simulink model "MATE_9LevelDrive_LowHarmonicRectifier"  (R2024b)
settings: Solver=FixedStepDiscrete  StartTime=0.0  StopTime=1  FixedStep=Ts  RelTol=1e-3
PostLoadFcn:
  | Ts=25e-6; initDrive9Level;Rsnu=30; Csnu=3e-6;Ron=0.01;Roff=1e6; Vf=2;
InitFcn:
  | Ts=25e-6; initDrive9Level;Rsnu=30; Csnu=3e-6;Ron=0.01;Roff=1e6; Vf=2;
values from neighbouring files (symbols this model uses):
  Lbase = Zbase/wbase    (= 0.0044902914611)    [initDrive9Level.m]
  Rgnd_rectifier = 1e4    (= 10000)    [initDrive9Level.m]
  T_2wind_ratio = 0.2677    [initDrive9Level.m]
  T_Lpu = Ltot_pu*9/10    (= 0.036)    [initDrive9Level.m]
  T_Lpu_pri = Ltot_pu/10    (= 0.004)    [initDrive9Level.m]
  T_Rpu = Rtot_pu*9/10    (= 0.009)    [initDrive9Level.m]
  T_Rpu_pri = Rtot_pu/10    (= 0.001)    [initDrive9Level.m]
  T_Vpri = 3000    [initDrive9Level.m]
  T_Vpri_15comp = 1.1168    [initDrive9Level.m]
  T_Vsec = 920    [initDrive9Level.m]
  Zbase = T_Vsec*T_Vsec/T_Pbase    (= 1.6928)    [initDrive9Level.m]
undefined symbols (not defined in the file or in its folder): DiscIntNeverNeededParam, gcbh, sps_rtmsupport
libraries: fl_lib x192, ee_lib x105, simetranss x26, nesl_utility x21
(part 4 of 5)

== system MATE_9LevelDrive_LowHarmonicRectifier/Diode Bridge with snubber2/RCsnuber2 ==
  Capacitor : fl_lib/Electrical/Electrical Elements/Capacitor  c=Csnu F  r=0 Ohm  g=0 1/Ohm  i_specify=off  i_priority=None  i=0 A  i_nominal_specify=off  i_nominal_value=1  i_nominal_unit=A  v_specify=off  v_priority=None  v=0 V  v_nominal_specify=off  v_nominal_value=1  v_nominal_unit=V  vc_specify=off  vc_priority=High  vc=0 V  vc_nominal_specify=off  vc_nominal_value=1  vc_nominal_unit=V
  Resistor : fl_lib/Electrical/Electrical Elements/Resistor  R=Rsnu Ohm  i_specify=off  i_priority=None  i=0 A  i_nominal_specify=off  i_nominal_value=1  i_nominal_unit=A  v_specify=off  v_priority=None  v=0 V  v_nominal_specify=off  v_nominal_value=1  v_nominal_unit=V
  + : PMIOPort  Side=Left
  - : PMIOPort  Port=2  Side=Right
  connections:
  Resistor/RConn1 -- -/RConn1
  Capacitor/LConn1 -- +/RConn1
  Resistor/LConn1 -- Capacitor/RConn1

== system MATE_9LevelDrive_LowHarmonicRectifier/Diode Bridge with snubber2/RCsnuber3 ==
  Capacitor : fl_lib/Electrical/Electrical Elements/Capacitor  c=Csnu F  r=0 Ohm  g=0 1/Ohm  i_specify=off  i_priority=None  i=0 A  i_nominal_specify=off  i_nominal_value=1  i_nominal_unit=A  v_specify=off  v_priority=None  v=0 V  v_nominal_specify=off  v_nominal_value=1  v_nominal_unit=V  vc_specify=off  vc_priority=High  vc=0 V  vc_nominal_specify=off  vc_nominal_value=1  vc_nominal_unit=V
  Resistor : fl_lib/Electrical/Electrical Elements/Resistor  R=Rsnu Ohm  i_specify=off  i_priority=None  i=0 A  i_nominal_specify=off  i_nominal_value=1  i_nominal_unit=A  v_specify=off  v_priority=None  v=0 V  v_nominal_specify=off  v_nominal_value=1  v_nominal_unit=V
  + : PMIOPort  Side=Left
  - : PMIOPort  Port=2  Side=Right
  connections:
  Resistor/LConn1 -- Capacitor/RConn1
  Capacitor/LConn1 -- +/RConn1
  Resistor/RConn1 -- -/RConn1

== system MATE_9LevelDrive_LowHarmonicRectifier/Diode Bridge with snubber2/RCsnuber4 ==
  Capacitor : fl_lib/Electrical/Electrical Elements/Capacitor  c=Csnu F  r=0 Ohm  g=0 1/Ohm  i_specify=off  i_priority=None  i=0 A  i_nominal_specify=off  i_nominal_value=1  i_nominal_unit=A  v_specify=off  v_priority=None  v=0 V  v_nominal_specify=off  v_nominal_value=1  v_nominal_unit=V  vc_specify=off  vc_priority=High  vc=0 V  vc_nominal_specify=off  vc_nominal_value=1  vc_nominal_unit=V
  Resistor : fl_lib/Electrical/Electrical Elements/Resistor  R=Rsnu Ohm  i_specify=off  i_priority=None  i=0 A  i_nominal_specify=off  i_nominal_value=1  i_nominal_unit=A  v_specify=off  v_priority=None  v=0 V  v_nominal_specify=off  v_nominal_value=1  v_nominal_unit=V
  + : PMIOPort  Side=Left
  - : PMIOPort  Port=2  Side=Right
  connections:
  Resistor/LConn1 -- Capacitor/RConn1
  Capacitor/LConn1 -- +/RConn1
  Resistor/RConn1 -- -/RConn1

== system MATE_9LevelDrive_LowHarmonicRectifier/Diode Bridge with snubber2/RCsnuber5 ==
  Capacitor : fl_lib/Electrical/Electrical Elements/Capacitor  c=Csnu F  r=0 Ohm  g=0 1/Ohm  i_specify=off  i_priority=None  i=0 A  i_nominal_specify=off  i_nominal_value=1  i_nominal_unit=A  v_specify=off  v_priority=None  v=0 V  v_nominal_specify=off  v_nominal_value=1  v_nominal_unit=V  vc_specify=off  vc_priority=High  vc=0 V  vc_nominal_specify=off  vc_nominal_value=1  vc_nominal_unit=V
  Resistor : fl_lib/Electrical/Electrical Elements/Resistor  R=Rsnu Ohm  i_specify=off  i_priority=None  i=0 A  i_nominal_specify=off  i_nominal_value=1  i_nominal_unit=A  v_specify=off  v_priority=None  v=0 V  v_nominal_specify=off  v_nominal_value=1  v_nominal_unit=V
  + : PMIOPort  Side=Left
  - : PMIOPort  Port=2  Side=Right
  connections:
  Resistor/RConn1 -- -/RConn1
  Capacitor/LConn1 -- +/RConn1
  Resistor/LConn1 -- Capacitor/RConn1

== system MATE_9LevelDrive_LowHarmonicRectifier/Diode Bridge with snubber3/RCsnuber ==
  Capacitor : fl_lib/Electrical/Electrical Elements/Capacitor  c=Csnu F  r=0 Ohm  g=0 1/Ohm  i_specify=off  i_priority=None  i=0 A  i_nominal_specify=off  i_nominal_value=1  i_nominal_unit=A  v_specify=off  v_priority=None  v=0 V  v_nominal_specify=off  v_nominal_value=1  v_nominal_unit=V  vc_specify=off  vc_priority=High  vc=0 V  vc_nominal_specify=off  vc_nominal_value=1  vc_nominal_unit=V
  Resistor : fl_lib/Electrical/Electrical Elements/Resistor  R=Rsnu Ohm  i_specify=off  i_priority=None  i=0 A  i_nominal_specify=off  i_nominal_value=1  i_nominal_unit=A  v_specify=off  v_priority=None  v=0 V  v_nominal_specify=off  v_nominal_value=1  v_nominal_unit=V
  + : PMIOPort  Side=Left
  - : PMIOPort  Port=2  Side=Right
  connections:
  Resistor/LConn1 -- Capacitor/RConn1
  Capacitor/LConn1 -- +/RConn1
  Resistor/RConn1 -- -/RConn1

== system MATE_9LevelDrive_LowHarmonicRectifier/Diode Bridge with snubber3/RCsnuber1 ==
  Capacitor : fl_lib/Electrical/Electrical Elements/Capacitor  c=Csnu F  r=0 Ohm  g=0 1/Ohm  i_specify=off  i_priority=None  i=0 A  i_nominal_specify=off  i_nominal_value=1  i_nominal_unit=A  v_specify=off  v_priority=None  v=0 V  v_nominal_specify=off  v_nominal_value=1  v_nominal_unit=V  vc_specify=off  vc_priority=High  vc=0 V  vc_nominal_specify=off  vc_nominal_value=1  vc_nominal_unit=V
  Resistor : fl_lib/Electrical/Electrical Elements/Resistor  R=Rsnu Ohm  i_specify=off  i_priority=None  i=0 A  i_nominal_specify=off  i_nominal_value=1  i_nominal_unit=A  v_specify=off  v_priority=None  v=0 V  v_nominal_specify=off  v_nominal_value=1  v_nominal_unit=V
  + : PMIOPort  Side=Left
  - : PMIOPort  Port=2  Side=Right
  connections:
  Resistor/RConn1 -- -/RConn1
  Capacitor/LConn1 -- +/RConn1
  Resistor/LConn1 -- Capacitor/RConn1

== system MATE_9LevelDrive_LowHarmonicRectifier/Diode Bridge with snubber3/RCsnuber2 ==
  Capacitor : fl_lib/Electrical/Electrical Elements/Capacitor  c=Csnu F  r=0 Ohm  g=0 1/Ohm  i_specify=off  i_priority=None  i=0 A  i_nominal_specify=off  i_nominal_value=1  i_nominal_unit=A  v_specify=off  v_priority=None  v=0 V  v_nominal_specify=off  v_nominal_value=1  v_nominal_unit=V  vc_specify=off  vc_priority=High  vc=0 V  vc_nominal_specify=off  vc_nominal_value=1  vc_nominal_unit=V
  Resistor : fl_lib/Electrical/Electrical Elements/Resistor  R=Rsnu Ohm  i_specify=off  i_priority=None  i=0 A  i_nominal_specify=off  i_nominal_value=1  i_nominal_unit=A  v_specify=off  v_priority=None  v=0 V  v_nominal_specify=off  v_nominal_value=1  v_nominal_unit=V
  + : PMIOPort  Side=Left
  - : PMIOPort  Port=2  Side=Right
  connections:
  Resistor/LConn1 -- Capacitor/RConn1
  Capacitor/LConn1 -- +/RConn1
  Resistor/RConn1 -- -/RConn1

== system MATE_9LevelDrive_LowHarmonicRectifier/Diode Bridge with snubber3/RCsnuber3 ==
  Capacitor : fl_lib/Electrical/Electrical Elements/Capacitor  c=Csnu F  r=0 Ohm  g=0 1/Ohm  i_specify=off  i_priority=None  i=0 A  i_nominal_specify=off  i_nominal_value=1  i_nominal_unit=A  v_specify=off  v_priority=None  v=0 V  v_nominal_specify=off  v_nominal_value=1  v_nominal_unit=V  vc_specify=off  vc_priority=High  vc=0 V  vc_nominal_specify=off  vc_nominal_value=1  vc_nominal_unit=V
  Resistor : fl_lib/Electrical/Electrical Elements/Resistor  R=Rsnu Ohm  i_specify=off  i_priority=None  i=0 A  i_nominal_specify=off  i_nominal_value=1  i_nominal_unit=A  v_specify=off  v_priority=None  v=0 V  v_nominal_specify=off  v_nominal_value=1  v_nominal_unit=V
  + : PMIOPort  Side=Left
  - : PMIOPort  Port=2  Side=Right
  connections:
  Resistor/RConn1 -- -/RConn1
  Capacitor/LConn1 -- +/RConn1
  Resistor/LConn1 -- Capacitor/RConn1

== system MATE_9LevelDrive_LowHarmonicRectifier/Diode Bridge with snubber3/RCsnuber4 ==
  Capacitor : fl_lib/Electrical/Electrical Elements/Capacitor  c=Csnu F  r=0 Ohm  g=0 1/Ohm  i_specify=off  i_priority=None  i=0 A  i_nominal_specify=off  i_nominal_value=1  i_nominal_unit=A  v_specify=off  v_priority=None  v=0 V  v_nominal_specify=off  v_nominal_value=1  v_nominal_unit=V  vc_specify=off  vc_priority=High  vc=0 V  vc_nominal_specify=off  vc_nominal_value=1  vc_nominal_unit=V
  Resistor : fl_lib/Electrical/Electrical Elements/Resistor  R=Rsnu Ohm  i_specify=off  i_priority=None  i=0 A  i_nominal_specify=off  i_nominal_value=1  i_nominal_unit=A  v_specify=off  v_priority=None  v=0 V  v_nominal_specify=off  v_nominal_value=1  v_nominal_unit=V
  + : PMIOPort  Side=Left
  - : PMIOPort  Port=2  Side=Right
  connections:
  Resistor/RConn1 -- -/RConn1
  Capacitor/LConn1 -- +/RConn1
  Resistor/LConn1 -- Capacitor/RConn1

== system MATE_9LevelDrive_LowHarmonicRectifier/Diode Bridge with snubber3/RCsnuber5 ==
  Capacitor : fl_lib/Electrical/Electrical Elements/Capacitor  c=Csnu F  r=0 Ohm  g=0 1/Ohm  i_specify=off  i_priority=None  i=0 A  i_nominal_specify=off  i_nominal_value=1  i_nominal_unit=A  v_specify=off  v_priority=None  v=0 V  v_nominal_specify=off  v_nominal_value=1  v_nominal_unit=V  vc_specify=off  vc_priority=High  vc=0 V  vc_nominal_specify=off  vc_nominal_value=1  vc_nominal_unit=V
  Resistor : fl_lib/Electrical/Electrical Elements/Resistor  R=Rsnu Ohm  i_specify=off  i_priority=None  i=0 A  i_nominal_specify=off  i_nominal_value=1  i_nominal_unit=A  v_specify=off  v_priority=None  v=0 V  v_nominal_specify=off  v_nominal_value=1  v_nominal_unit=V
  + : PMIOPort  Side=Left
  - : PMIOPort  Port=2  Side=Right
  connections:
  Resistor/LConn1 -- Capacitor/RConn1
  Capacitor/LConn1 -- +/RConn1
  Resistor/RConn1 -- -/RConn1

== system MATE_9LevelDrive_LowHarmonicRectifier/Diode Bridge with snubber4/RCsnuber ==
  Capacitor : fl_lib/Electrical/Electrical Elements/Capacitor  c=Csnu F  r=0 Ohm  g=0 1/Ohm  i_specify=off  i_priority=None  i=0 A  i_nominal_specify=off  i_nominal_value=1  i_nominal_unit=A  v_specify=off  v_priority=None  v=0 V  v_nominal_specify=off  v_nominal_value=1  v_nominal_unit=V  vc_specify=off  vc_priority=High  vc=0 V  vc_nominal_specify=off  vc_nominal_value=1  vc_nominal_unit=V
  Resistor : fl_lib/Electrical/Electrical Elements/Resistor  R=Rsnu Ohm  i_specify=off  i_priority=None  i=0 A  i_nominal_specify=off  i_nominal_value=1  i_nominal_unit=A  v_specify=off  v_priority=None  v=0 V  v_nominal_specify=off  v_nominal_value=1  v_nominal_unit=V
  + : PMIOPort  Side=Left
  - : PMIOPort  Port=2  Side=Right
  connections:
  Resistor/RConn1 -- -/RConn1
  Capacitor/LConn1 -- +/RConn1
  Resistor/LConn1 -- Capacitor/RConn1

== system MATE_9LevelDrive_LowHarmonicRectifier/Diode Bridge with snubber4/RCsnuber1 ==
  Capacitor : fl_lib/Electrical/Electrical Elements/Capacitor  c=Csnu F  r=0 Ohm  g=0 1/Ohm  i_specify=off  i_priority=None  i=0 A  i_nominal_specify=off  i_nominal_value=1  i_nominal_unit=A  v_specify=off  v_priority=None  v=0 V  v_nominal_specify=off  v_nominal_value=1  v_nominal_unit=V  vc_specify=off  vc_priority=High  vc=0 V  vc_nominal_specify=off  vc_nominal_value=1  vc_nominal_unit=V
  Resistor : fl_lib/Electrical/Electrical Elements/Resistor  R=Rsnu Ohm  i_specify=off  i_priority=None  i=0 A  i_nominal_specify=off  i_nominal_value=1  i_nominal_unit=A  v_specify=off  v_priority=None  v=0 V  v_nominal_specify=off  v_nominal_value=1  v_nominal_unit=V
  + : PMIOPort  Side=Left
  - : PMIOPort  Port=2  Side=Right
  connections:
  Resistor/LConn1 -- Capacitor/RConn1
  Capacitor/LConn1 -- +/RConn1
  Resistor/RConn1 -- -/RConn1

== system MATE_9LevelDrive_LowHarmonicRectifier/Diode Bridge with snubber4/RCsnuber2 ==
  Capacitor : fl_lib/Electrical/Electrical Elements/Capacitor  c=Csnu F  r=0 Ohm  g=0 1/Ohm  i_specify=off  i_priority=None  i=0 A  i_nominal_specify=off  i_nominal_value=1  i_nominal_unit=A  v_specify=off  v_priority=None  v=0 V  v_nominal_specify=off  v_nominal_value=1  v_nominal_unit=V  vc_specify=off  vc_priority=High  vc=0 V  vc_nominal_specify=off  vc_nominal_value=1  vc_nominal_unit=V
  Resistor : fl_lib/Electrical/Electrical Elements/Resistor  R=Rsnu Ohm  i_specify=off  i_priority=None  i=0 A  i_nominal_specify=off  i_nominal_value=1  i_nominal_unit=A  v_specify=off  v_priority=None  v=0 V  v_nominal_specify=off  v_nominal_value=1  v_nominal_unit=V
  + : PMIOPort  Side=Left
  - : PMIOPort  Port=2  Side=Right
  connections:
  Resistor/RConn1 -- -/RConn1
  Capacitor/LConn1 -- +/RConn1
  Resistor/LConn1 -- Capacitor/RConn1

== system MATE_9LevelDrive_LowHarmonicRectifier/Diode Bridge with snubber4/RCsnuber3 ==
  Capacitor : fl_lib/Electrical/Electrical Elements/Capacitor  c=Csnu F  r=0 Ohm  g=0 1/Ohm  i_specify=off  i_priority=None  i=0 A  i_nominal_specify=off  i_nominal_value=1  i_nominal_unit=A  v_specify=off  v_priority=None  v=0 V  v_nominal_specify=off  v_nominal_value=1  v_nominal_unit=V  vc_specify=off  vc_priority=High  vc=0 V  vc_nominal_specify=off  vc_nominal_value=1  vc_nominal_unit=V
  Resistor : fl_lib/Electrical/Electrical Elements/Resistor  R=Rsnu Ohm  i_specify=off  i_priority=None  i=0 A  i_nominal_specify=off  i_nominal_value=1  i_nominal_unit=A  v_specify=off  v_priority=None  v=0 V  v_nominal_specify=off  v_nominal_value=1  v_nominal_unit=V
  + : PMIOPort  Side=Left
  - : PMIOPort  Port=2  Side=Right
  connections:
  Resistor/LConn1 -- Capacitor/RConn1
  Capacitor/LConn1 -- +/RConn1
  Resistor/RConn1 -- -/RConn1

== system MATE_9LevelDrive_LowHarmonicRectifier/Diode Bridge with snubber4/RCsnuber4 ==
  Capacitor : fl_lib/Electrical/Electrical Elements/Capacitor  c=Csnu F  r=0 Ohm  g=0 1/Ohm  i_specify=off  i_priority=None  i=0 A  i_nominal_specify=off  i_nominal_value=1  i_nominal_unit=A  v_specify=off  v_priority=None  v=0 V  v_nominal_specify=off  v_nominal_value=1  v_nominal_unit=V  vc_specify=off  vc_priority=High  vc=0 V  vc_nominal_specify=off  vc_nominal_value=1  vc_nominal_unit=V
  Resistor : fl_lib/Electrical/Electrical Elements/Resistor  R=Rsnu Ohm  i_specify=off  i_priority=None  i=0 A  i_nominal_specify=off  i_nominal_value=1  i_nominal_unit=A  v_specify=off  v_priority=None  v=0 V  v_nominal_specify=off  v_nominal_value=1  v_nominal_unit=V
  + : PMIOPort  Side=Left
  - : PMIOPort  Port=2  Side=Right
  connections:
  Resistor/LConn1 -- Capacitor/RConn1
  Capacitor/LConn1 -- +/RConn1
  Resistor/RConn1 -- -/RConn1

== system MATE_9LevelDrive_LowHarmonicRectifier/Diode Bridge with snubber4/RCsnuber5 ==
  Capacitor : fl_lib/Electrical/Electrical Elements/Capacitor  c=Csnu F  r=0 Ohm  g=0 1/Ohm  i_specify=off  i_priority=None  i=0 A  i_nominal_specify=off  i_nominal_value=1  i_nominal_unit=A  v_specify=off  v_priority=None  v=0 V  v_nominal_specify=off  v_nominal_value=1  v_nominal_unit=V  vc_specify=off  vc_priority=High  vc=0 V  vc_nominal_specify=off  vc_nominal_value=1  vc_nominal_unit=V
  Resistor : fl_lib/Electrical/Electrical Elements/Resistor  R=Rsnu Ohm  i_specify=off  i_priority=None  i=0 A  i_nominal_specify=off  i_nominal_value=1  i_nominal_unit=A  v_specify=off  v_priority=None  v=0 V  v_nominal_specify=off  v_nominal_value=1  v_nominal_unit=V
  + : PMIOPort  Side=Left
  - : PMIOPort  Port=2  Side=Right
  connections:
  Resistor/RConn1 -- -/RConn1
  Capacitor/LConn1 -- +/RConn1
  Resistor/LConn1 -- Capacitor/RConn1

== system MATE_9LevelDrive_LowHarmonicRectifier/Diode Bridge with snubber5/RCsnuber ==
  Capacitor : fl_lib/Electrical/Electrical Elements/Capacitor  c=Csnu F  r=0 Ohm  g=0 1/Ohm  i_specify=off  i_priority=None  i=0 A  i_nominal_specify=off  i_nominal_value=1  i_nominal_unit=A  v_specify=off  v_priority=None  v=0 V  v_nominal_specify=off  v_nominal_value=1  v_nominal_unit=V  vc_specify=off  vc_priority=High  vc=0 V  vc_nominal_specify=off  vc_nominal_value=1  vc_nominal_unit=V
  Resistor : fl_lib/Electrical/Electrical Elements/Resistor  R=Rsnu Ohm  i_specify=off  i_priority=None  i=0 A  i_nominal_specify=off  i_nominal_value=1  i_nominal_unit=A  v_specify=off  v_priority=None  v=0 V  v_nominal_specify=off  v_nominal_value=1  v_nominal_unit=V
  + : PMIOPort  Side=Left
  - : PMIOPort  Port=2  Side=Right
  connections:
  Resistor/LConn1 -- Capacitor/RConn1
  Capacitor/LConn1 -- +/RConn1
  Resistor/RConn1 -- -/RConn1

== system MATE_9LevelDrive_LowHarmonicRectifier/Diode Bridge with snubber5/RCsnuber1 ==
  Capacitor : fl_lib/Electrical/Electrical Elements/Capacitor  c=Csnu F  r=0 Ohm  g=0 1/Ohm  i_specify=off  i_priority=None  i=0 A  i_nominal_specify=off  i_nominal_value=1  i_nominal_unit=A  v_specify=off  v_priority=None  v=0 V  v_nominal_specify=off  v_nominal_value=1  v_nominal_unit=V  vc_specify=off  vc_priority=High  vc=0 V  vc_nominal_specify=off  vc_nominal_value=1  vc_nominal_unit=V
  Resistor : fl_lib/Electrical/Electrical Elements/Resistor  R=Rsnu Ohm  i_specify=off  i_priority=None  i=0 A  i_nominal_specify=off  i_nominal_value=1  i_nominal_unit=A  v_specify=off  v_priority=None  v=0 V  v_nominal_specify=off  v_nominal_value=1  v_nominal_unit=V
  + : PMIOPort  Side=Left
  - : PMIOPort  Port=2  Side=Right
  connections:
  Resistor/RConn1 -- -/RConn1
  Capacitor/LConn1 -- +/RConn1
  Resistor/LConn1 -- Capacitor/RConn1

== system MATE_9LevelDrive_LowHarmonicRectifier/Diode Bridge with snubber5/RCsnuber2 ==
  Capacitor : fl_lib/Electrical/Electrical Elements/Capacitor  c=Csnu F  r=0 Ohm  g=0 1/Ohm  i_specify=off  i_priority=None  i=0 A  i_nominal_specify=off  i_nominal_value=1  i_nominal_unit=A  v_specify=off  v_priority=None  v=0 V  v_nominal_specify=off  v_nominal_value=1  v_nominal_unit=V  vc_specify=off  vc_priority=High  vc=0 V  vc_nominal_specify=off  vc_nominal_value=1  vc_nominal_unit=V
  Resistor : fl_lib/Electrical/Electrical Elements/Resistor  R=Rsnu Ohm  i_specify=off  i_priority=None  i=0 A  i_nominal_specify=off  i_nominal_value=1  i_nominal_unit=A  v_specify=off  v_priority=None  v=0 V  v_nominal_specify=off  v_nominal_value=1  v_nominal_unit=V
  + : PMIOPort  Side=Left
  - : PMIOPort  Port=2  Side=Right
  connections:
  Resistor/LConn1 -- Capacitor/RConn1
  Capacitor/LConn1 -- +/RConn1
  Resistor/RConn1 -- -/RConn1

== system MATE_9LevelDrive_LowHarmonicRectifier/Diode Bridge with snubber5/RCsnuber3 ==
  Capacitor : fl_lib/Electrical/Electrical Elements/Capacitor  c=Csnu F  r=0 Ohm  g=0 1/Ohm  i_specify=off  i_priority=None  i=0 A  i_nominal_specify=off  i_nominal_value=1  i_nominal_unit=A  v_specify=off  v_priority=None  v=0 V  v_nominal_specify=off  v_nominal_value=1  v_nominal_unit=V  vc_specify=off  vc_priority=High  vc=0 V  vc_nominal_specify=off  vc_nominal_value=1  vc_nominal_unit=V
  Resistor : fl_lib/Electrical/Electrical Elements/Resistor  R=Rsnu Ohm  i_specify=off  i_priority=None  i=0 A  i_nominal_specify=off  i_nominal_value=1  i_nominal_unit=A  v_specify=off  v_priority=None  v=0 V  v_nominal_specify=off  v_nominal_value=1  v_nominal_unit=V
  + : PMIOPort  Side=Left
  - : PMIOPort  Port=2  Side=Right
  connections:
  Resistor/RConn1 -- -/RConn1
  Capacitor/LConn1 -- +/RConn1
  Resistor/LConn1 -- Capacitor/RConn1

== system MATE_9LevelDrive_LowHarmonicRectifier/Diode Bridge with snubber5/RCsnuber4 ==
  Capacitor : fl_lib/Electrical/Electrical Elements/Capacitor  c=Csnu F  r=0 Ohm  g=0 1/Ohm  i_specify=off  i_priority=None  i=0 A  i_nominal_specify=off  i_nominal_value=1  i_nominal_unit=A  v_specify=off  v_priority=None  v=0 V  v_nominal_specify=off  v_nominal_value=1  v_nominal_unit=V  vc_specify=off  vc_priority=High  vc=0 V  vc_nominal_specify=off  vc_nominal_value=1  vc_nominal_unit=V
  Resistor : fl_lib/Electrical/Electrical Elements/Resistor  R=Rsnu Ohm  i_specify=off  i_priority=None  i=0 A  i_nominal_specify=off  i_nominal_value=1  i_nominal_unit=A  v_specify=off  v_priority=None  v=0 V  v_nominal_specify=off  v_nominal_value=1  v_nominal_unit=V
  + : PMIOPort  Side=Left
  - : PMIOPort  Port=2  Side=Right
  connections:
  Resistor/RConn1 -- -/RConn1
  Capacitor/LConn1 -- +/RConn1
  Resistor/LConn1 -- Capacitor/RConn1

== system MATE_9LevelDrive_LowHarmonicRectifier/Diode Bridge with snubber5/RCsnuber5 ==
  Capacitor : fl_lib/Electrical/Electrical Elements/Capacitor  c=Csnu F  r=0 Ohm  g=0 1/Ohm  i_specify=off  i_priority=None  i=0 A  i_nominal_specify=off  i_nominal_value=1  i_nominal_unit=A  v_specify=off  v_priority=None  v=0 V  v_nominal_specify=off  v_nominal_value=1  v_nominal_unit=V  vc_specify=off  vc_priority=High  vc=0 V  vc_nominal_specify=off  vc_nominal_value=1  vc_nominal_unit=V
  Resistor : fl_lib/Electrical/Electrical Elements/Resistor  R=Rsnu Ohm  i_specify=off  i_priority=None  i=0 A  i_nominal_specify=off  i_nominal_value=1  i_nominal_unit=A  v_specify=off  v_priority=None  v=0 V  v_nominal_specify=off  v_nominal_value=1  v_nominal_unit=V
  + : PMIOPort  Side=Left
  - : PMIOPort  Port=2  Side=Right
  connections:
  Resistor/LConn1 -- Capacitor/RConn1
  Capacitor/LConn1 -- +/RConn1
  Resistor/RConn1 -- -/RConn1

== system MATE_9LevelDrive_LowHarmonicRectifier/Diode Bridge with snubber6/RCsnuber ==
  Capacitor : fl_lib/Electrical/Electrical Elements/Capacitor  c=Csnu F  r=0 Ohm  g=0 1/Ohm  i_specify=off  i_priority=None  i=0 A  i_nominal_specify=off  i_nominal_value=1  i_nominal_unit=A  v_specify=off  v_priority=None  v=0 V  v_nominal_specify=off  v_nominal_value=1  v_nominal_unit=V  vc_specify=off  vc_priority=High  vc=0 V  vc_nominal_specify=off  vc_nominal_value=1  vc_nominal_unit=V
  Resistor : fl_lib/Electrical/Electrical Elements/Resistor  R=Rsnu Ohm  i_specify=off  i_priority=None  i=0 A  i_nominal_specify=off  i_nominal_value=1  i_nominal_unit=A  v_specify=off  v_priority=None  v=0 V  v_nominal_specify=off  v_nominal_value=1  v_nominal_unit=V
  + : PMIOPort  Side=Left
  - : PMIOPort  Port=2  Side=Right
  connections:
  Resistor/RConn1 -- -/RConn1
  Capacitor/LConn1 -- +/RConn1
  Resistor/LConn1 -- Capacitor/RConn1

== system MATE_9LevelDrive_LowHarmonicRectifier/Diode Bridge with snubber6/RCsnuber1 ==
  Capacitor : fl_lib/Electrical/Electrical Elements/Capacitor  c=Csnu F  r=0 Ohm  g=0 1/Ohm  i_specify=off  i_priority=None  i=0 A  i_nominal_specify=off  i_nominal_value=1  i_nominal_unit=A  v_specify=off  v_priority=None  v=0 V  v_nominal_specify=off  v_nominal_value=1  v_nominal_unit=V  vc_specify=off  vc_priority=High  vc=0 V  vc_nominal_specify=off  vc_nominal_value=1  vc_nominal_unit=V
  Resistor : fl_lib/Electrical/Electrical Elements/Resistor  R=Rsnu Ohm  i_specify=off  i_priority=None  i=0 A  i_nominal_specify=off  i_nominal_value=1  i_nominal_unit=A  v_specify=off  v_priority=None  v=0 V  v_nominal_specify=off  v_nominal_value=1  v_nominal_unit=V
  + : PMIOPort  Side=Left
  - : PMIOPort  Port=2  Side=Right
  connections:
  Resistor/LConn1 -- Capacitor/RConn1
  Capacitor/LConn1 -- +/RConn1
  Resistor/RConn1 -- -/RConn1

== system MATE_9LevelDrive_LowHarmonicRectifier/Diode Bridge with snubber6/RCsnuber2 ==
  Capacitor : fl_lib/Electrical/Electrical Elements/Capacitor  c=Csnu F  r=0 Ohm  g=0 1/Ohm  i_specify=off  i_priority=None  i=0 A  i_nominal_specify=off  i_nominal_value=1  i_nominal_unit=A  v_specify=off  v_priority=None  v=0 V  v_nominal_specify=off  v_nominal_value=1  v_nominal_unit=V  vc_specify=off  vc_priority=High  vc=0 V  vc_nominal_specify=off  vc_nominal_value=1  vc_nominal_unit=V
  Resistor : fl_lib/Electrical/Electrical Elements/Resistor  R=Rsnu Ohm  i_specify=off  i_priority=None  i=0 A  i_nominal_specify=off  i_nominal_value=1  i_nominal_unit=A  v_specify=off  v_priority=None  v=0 V  v_nominal_specify=off  v_nominal_value=1  v_nominal_unit=V
  + : PMIOPort  Side=Left
  - : PMIOPort  Port=2  Side=Right
  connections:
  Resistor/RConn1 -- -/RConn1
  Capacitor/LConn1 -- +/RConn1
  Resistor/LConn1 -- Capacitor/RConn1

== system MATE_9LevelDrive_LowHarmonicRectifier/Diode Bridge with snubber6/RCsnuber3 ==
  Capacitor : fl_lib/Electrical/Electrical Elements/Capacitor  c=Csnu F  r=0 Ohm  g=0 1/Ohm  i_specify=off  i_priority=None  i=0 A  i_nominal_specify=off  i_nominal_value=1  i_nominal_unit=A  v_specify=off  v_priority=None  v=0 V  v_nominal_specify=off  v_nominal_value=1  v_nominal_unit=V  vc_specify=off  vc_priority=High  vc=0 V  vc_nominal_specify=off  vc_nominal_value=1  vc_nominal_unit=V
  Resistor : fl_lib/Electrical/Electrical Elements/Resistor  R=Rsnu Ohm  i_specify=off  i_priority=None  i=0 A  i_nominal_specify=off  i_nominal_value=1  i_nominal_unit=A  v_specify=off  v_priority=None  v=0 V  v_nominal_specify=off  v_nominal_value=1  v_nominal_unit=V
  + : PMIOPort  Side=Left
  - : PMIOPort  Port=2  Side=Right
  connections:
  Resistor/LConn1 -- Capacitor/RConn1
  Capacitor/LConn1 -- +/RConn1
  Resistor/RConn1 -- -/RConn1

== system MATE_9LevelDrive_LowHarmonicRectifier/Diode Bridge with snubber6/RCsnuber4 ==
  Capacitor : fl_lib/Electrical/Electrical Elements/Capacitor  c=Csnu F  r=0 Ohm  g=0 1/Ohm  i_specify=off  i_priority=None  i=0 A  i_nominal_specify=off  i_nominal_value=1  i_nominal_unit=A  v_specify=off  v_priority=None  v=0 V  v_nominal_specify=off  v_nominal_value=1  v_nominal_unit=V  vc_specify=off  vc_priority=High  vc=0 V  vc_nominal_specify=off  vc_nominal_value=1  vc_nominal_unit=V
  Resistor : fl_lib/Electrical/Electrical Elements/Resistor  R=Rsnu Ohm  i_specify=off  i_priority=None  i=0 A  i_nominal_specify=off  i_nominal_value=1  i_nominal_unit=A  v_specify=off  v_priority=None  v=0 V  v_nominal_specify=off  v_nominal_value=1  v_nominal_unit=V
  + : PMIOPort  Side=Left
  - : PMIOPort  Port=2  Side=Right
  connections:
  Resistor/LConn1 -- Capacitor/RConn1
  Capacitor/LConn1 -- +/RConn1
  Resistor/RConn1 -- -/RConn1

== system MATE_9LevelDrive_LowHarmonicRectifier/Diode Bridge with snubber6/RCsnuber5 ==
  Capacitor : fl_lib/Electrical/Electrical Elements/Capacitor  c=Csnu F  r=0 Ohm  g=0 1/Ohm  i_specify=off  i_priority=None  i=0 A  i_nominal_specify=off  i_nominal_value=1  i_nominal_unit=A  v_specify=off  v_priority=None  v=0 V  v_nominal_specify=off  v_nominal_value=1  v_nominal_unit=V  vc_specify=off  vc_priority=High  vc=0 V  vc_nominal_specify=off  vc_nominal_value=1  vc_nominal_unit=V
  Resistor : fl_lib/Electrical/Electrical Elements/Resistor  R=Rsnu Ohm  i_specify=off  i_priority=None  i=0 A  i_nominal_specify=off  i_nominal_value=1  i_nominal_unit=A  v_specify=off  v_priority=None  v=0 V  v_nominal_specify=off  v_nominal_value=1  v_nominal_unit=V
  + : PMIOPort  Side=Left
  - : PMIOPort  Port=2  Side=Right
  connections:
  Resistor/RConn1 -- -/RConn1
  Capacitor/LConn1 -- +/RConn1
  Resistor/LConn1 -- Capacitor/RConn1

== system MATE_9LevelDrive_LowHarmonicRectifier/Diode Bridge with snubber7/RCsnuber ==
  Capacitor : fl_lib/Electrical/Electrical Elements/Capacitor  c=Csnu F  r=0 Ohm  g=0 1/Ohm  i_specify=off  i_priority=None  i=0 A  i_nominal_specify=off  i_nominal_value=1  i_nominal_unit=A  v_specify=off  v_priority=None  v=0 V  v_nominal_specify=off  v_nominal_value=1  v_nominal_unit=V  vc_specify=off  vc_priority=High  vc=0 V  vc_nominal_specify=off  vc_nominal_value=1  vc_nominal_unit=V
  Resistor : fl_lib/Electrical/Electrical Elements/Resistor  R=Rsnu Ohm  i_specify=off  i_priority=None  i=0 A  i_nominal_specify=off  i_nominal_value=1  i_nominal_unit=A  v_specify=off  v_priority=None  v=0 V  v_nominal_specify=off  v_nominal_value=1  v_nominal_unit=V
  + : PMIOPort  Side=Left
  - : PMIOPort  Port=2  Side=Right
  connections:
  Resistor/LConn1 -- Capacitor/RConn1
  Capacitor/LConn1 -- +/RConn1
  Resistor/RConn1 -- -/RConn1

== system MATE_9LevelDrive_LowHarmonicRectifier/Diode Bridge with snubber7/RCsnuber1 ==
  Capacitor : fl_lib/Electrical/Electrical Elements/Capacitor  c=Csnu F  r=0 Ohm  g=0 1/Ohm  i_specify=off  i_priority=None  i=0 A  i_nominal_specify=off  i_nominal_value=1  i_nominal_unit=A  v_specify=off  v_priority=None  v=0 V  v_nominal_specify=off  v_nominal_value=1  v_nominal_unit=V  vc_specify=off  vc_priority=High  vc=0 V  vc_nominal_specify=off  vc_nominal_value=1  vc_nominal_unit=V
  Resistor : fl_lib/Electrical/Electrical Elements/Resistor  R=Rsnu Ohm  i_specify=off  i_priority=None  i=0 A  i_nominal_specify=off  i_nominal_value=1  i_nominal_unit=A  v_specify=off  v_priority=None  v=0 V  v_nominal_specify=off  v_nominal_value=1  v_nominal_unit=V
  + : PMIOPort  Side=Left
  - : PMIOPort  Port=2  Side=Right
  connections:
  Resistor/RConn1 -- -/RConn1
  Capacitor/LConn1 -- +/RConn1
  Resistor/LConn1 -- Capacitor/RConn1

== system MATE_9LevelDrive_LowHarmonicRectifier/Diode Bridge with snubber7/RCsnuber2 ==
  Capacitor : fl_lib/Electrical/Electrical Elements/Capacitor  c=Csnu F  r=0 Ohm  g=0 1/Ohm  i_specify=off  i_priority=None  i=0 A  i_nominal_specify=off  i_nominal_value=1  i_nominal_unit=A  v_specify=off  v_priority=None  v=0 V  v_nominal_specify=off  v_nominal_value=1  v_nominal_unit=V  vc_specify=off  vc_priority=High  vc=0 V  vc_nominal_specify=off  vc_nominal_value=1  vc_nominal_unit=V
  Resistor : fl_lib/Electrical/Electrical Elements/Resistor  R=Rsnu Ohm  i_specify=off  i_priority=None  i=0 A  i_nominal_specify=off  i_nominal_value=1  i_nominal_unit=A  v_specify=off  v_priority=None  v=0 V  v_nominal_specify=off  v_nominal_value=1  v_nominal_unit=V
  + : PMIOPort  Side=Left
  - : PMIOPort  Port=2  Side=Right
  connections:
  Resistor/LConn1 -- Capacitor/RConn1
  Capacitor/LConn1 -- +/RConn1
  Resistor/RConn1 -- -/RConn1

== system MATE_9LevelDrive_LowHarmonicRectifier/Diode Bridge with snubber7/RCsnuber3 ==
  Capacitor : fl_lib/Electrical/Electrical Elements/Capacitor  c=Csnu F  r=0 Ohm  g=0 1/Ohm  i_specify=off  i_priority=None  i=0 A  i_nominal_specify=off  i_nominal_value=1  i_nominal_unit=A  v_specify=off  v_priority=None  v=0 V  v_nominal_specify=off  v_nominal_value=1  v_nominal_unit=V  vc_specify=off  vc_priority=High  vc=0 V  vc_nominal_specify=off  vc_nominal_value=1  vc_nominal_unit=V
  Resistor : fl_lib/Electrical/Electrical Elements/Resistor  R=Rsnu Ohm  i_specify=off  i_priority=None  i=0 A  i_nominal_specify=off  i_nominal_value=1  i_nominal_unit=A  v_specify=off  v_priority=None  v=0 V  v_nominal_specify=off  v_nominal_value=1  v_nominal_unit=V
  + : PMIOPort  Side=Left
  - : PMIOPort  Port=2  Side=Right
  connections:
  Resistor/RConn1 -- -/RConn1
  Capacitor/LConn1 -- +/RConn1
  Resistor/LConn1 -- Capacitor/RConn1

== system MATE_9LevelDrive_LowHarmonicRectifier/Diode Bridge with snubber7/RCsnuber4 ==
  Capacitor : fl_lib/Electrical/Electrical Elements/Capacitor  c=Csnu F  r=0 Ohm  g=0 1/Ohm  i_specify=off  i_priority=None  i=0 A  i_nominal_specify=off  i_nominal_value=1  i_nominal_unit=A  v_specify=off  v_priority=None  v=0 V  v_nominal_specify=off  v_nominal_value=1  v_nominal_unit=V  vc_specify=off  vc_priority=High  vc=0 V  vc_nominal_specify=off  vc_nominal_value=1  vc_nominal_unit=V
  Resistor : fl_lib/Electrical/Electrical Elements/Resistor  R=Rsnu Ohm  i_specify=off  i_priority=None  i=0 A  i_nominal_specify=off  i_nominal_value=1  i_nominal_unit=A  v_specify=off  v_priority=None  v=0 V  v_nominal_specify=off  v_nominal_value=1  v_nominal_unit=V
  + : PMIOPort  Side=Left
  - : PMIOPort  Port=2  Side=Right
  connections:
  Resistor/RConn1 -- -/RConn1
  Capacitor/LConn1 -- +/RConn1
  Resistor/LConn1 -- Capacitor/RConn1

== system MATE_9LevelDrive_LowHarmonicRectifier/Diode Bridge with snubber7/RCsnuber5 ==
  Capacitor : fl_lib/Electrical/Electrical Elements/Capacitor  c=Csnu F  r=0 Ohm  g=0 1/Ohm  i_specify=off  i_priority=None  i=0 A  i_nominal_specify=off  i_nominal_value=1  i_nominal_unit=A  v_specify=off  v_priority=None  v=0 V  v_nominal_specify=off  v_nominal_value=1  v_nominal_unit=V  vc_specify=off  vc_priority=High  vc=0 V  vc_nominal_specify=off  vc_nominal_value=1  vc_nominal_unit=V
  Resistor : fl_lib/Electrical/Electrical Elements/Resistor  R=Rsnu Ohm  i_specify=off  i_priority=None  i=0 A  i_nominal_specify=off  i_nominal_value=1  i_nominal_unit=A  v_specify=off  v_priority=None  v=0 V  v_nominal_specify=off  v_nominal_value=1  v_nominal_unit=V
  + : PMIOPort  Side=Left
  - : PMIOPort  Port=2  Side=Right
  connections:
  Resistor/LConn1 -- Capacitor/RConn1
  Capacitor/LConn1 -- +/RConn1
  Resistor/RConn1 -- -/RConn1

== system MATE_9LevelDrive_LowHarmonicRectifier/Diode Bridge with snubber8/RCsnuber ==
  Capacitor : fl_lib/Electrical/Electrical Elements/Capacitor  c=Csnu F  r=0 Ohm  g=0 1/Ohm  i_specify=off  i_priority=None  i=0 A  i_nominal_specify=off  i_nominal_value=1  i_nominal_unit=A  v_specify=off  v_priority=None  v=0 V  v_nominal_specify=off  v_nominal_value=1  v_nominal_unit=V  vc_specify=off  vc_priority=High  vc=0 V  vc_nominal_specify=off  vc_nominal_value=1  vc_nominal_unit=V
  Resistor : fl_lib/Electrical/Electrical Elements/Resistor  R=Rsnu Ohm  i_specify=off  i_priority=None  i=0 A  i_nominal_specify=off  i_nominal_value=1  i_nominal_unit=A  v_specify=off  v_priority=None  v=0 V  v_nominal_specify=off  v_nominal_value=1  v_nominal_unit=V
  + : PMIOPort  Side=Left
  - : PMIOPort  Port=2  Side=Right
  connections:
  Resistor/RConn1 -- -/RConn1
  Capacitor/LConn1 -- +/RConn1
  Resistor/LConn1 -- Capacitor/RConn1

== system MATE_9LevelDrive_LowHarmonicRectifier/Diode Bridge with snubber8/RCsnuber1 ==
  Capacitor : fl_lib/Electrical/Electrical Elements/Capacitor  c=Csnu F  r=0 Ohm  g=0 1/Ohm  i_specify=off  i_priority=None  i=0 A  i_nominal_specify=off  i_nominal_value=1  i_nominal_unit=A  v_specify=off  v_priority=None  v=0 V  v_nominal_specify=off  v_nominal_value=1  v_nominal_unit=V  vc_specify=off  vc_priority=High  vc=0 V  vc_nominal_specify=off  vc_nominal_value=1  vc_nominal_unit=V
  Resistor : fl_lib/Electrical/Electrical Elements/Resistor  R=Rsnu Ohm  i_specify=off  i_priority=None  i=0 A  i_nominal_specify=off  i_nominal_value=1  i_nominal_unit=A  v_specify=off  v_priority=None  v=0 V  v_nominal_specify=off  v_nominal_value=1  v_nominal_unit=V
  + : PMIOPort  Side=Left
  - : PMIOPort  Port=2  Side=Right
  connections:
  Resistor/LConn1 -- Capacitor/RConn1
  Capacitor/LConn1 -- +/RConn1
  Resistor/RConn1 -- -/RConn1

== system MATE_9LevelDrive_LowHarmonicRectifier/Diode Bridge with snubber8/RCsnuber2 ==
  Capacitor : fl_lib/Electrical/Electrical Elements/Capacitor  c=Csnu F  r=0 Ohm  g=0 1/Ohm  i_specify=off  i_priority=None  i=0 A  i_nominal_specify=off  i_nominal_value=1  i_nominal_unit=A  v_specify=off  v_priority=None  v=0 V  v_nominal_specify=off  v_nominal_value=1  v_nominal_unit=V  vc_specify=off  vc_priority=High  vc=0 V  vc_nominal_specify=off  vc_nominal_value=1  vc_nominal_unit=V
  Resistor : fl_lib/Electrical/Electrical Elements/Resistor  R=Rsnu Ohm  i_specify=off  i_priority=None  i=0 A  i_nominal_specify=off  i_nominal_value=1  i_nominal_unit=A  v_specify=off  v_priority=None  v=0 V  v_nominal_specify=off  v_nominal_value=1  v_nominal_unit=V
  + : PMIOPort  Side=Left
  - : PMIOPort  Port=2  Side=Right
  connections:
  Resistor/RConn1 -- -/RConn1
  Capacitor/LConn1 -- +/RConn1
  Resistor/LConn1 -- Capacitor/RConn1

== system MATE_9LevelDrive_LowHarmonicRectifier/Diode Bridge with snubber8/RCsnuber3 ==
  Capacitor : fl_lib/Electrical/Electrical Elements/Capacitor  c=Csnu F  r=0 Ohm  g=0 1/Ohm  i_specify=off  i_priority=None  i=0 A  i_nominal_specify=off  i_nominal_value=1  i_nominal_unit=A  v_specify=off  v_priority=None  v=0 V  v_nominal_specify=off  v_nominal_value=1  v_nominal_unit=V  vc_specify=off  vc_priority=High  vc=0 V  vc_nominal_specify=off  vc_nominal_value=1  vc_nominal_unit=V
  Resistor : fl_lib/Electrical/Electrical Elements/Resistor  R=Rsnu Ohm  i_specify=off  i_priority=None  i=0 A  i_nominal_specify=off  i_nominal_value=1  i_nominal_unit=A  v_specify=off  v_priority=None  v=0 V  v_nominal_specify=off  v_nominal_value=1  v_nominal_unit=V
  + : PMIOPort  Side=Left
  - : PMIOPort  Port=2  Side=Right
  connections:
  Resistor/LConn1 -- Capacitor/RConn1
  Capacitor/LConn1 -- +/RConn1
  Resistor/RConn1 -- -/RConn1

== system MATE_9LevelDrive_LowHarmonicRectifier/Diode Bridge with snubber8/RCsnuber4 ==
  Capacitor : fl_lib/Electrical/Electrical Elements/Capacitor  c=Csnu F  r=0 Ohm  g=0 1/Ohm  i_specify=off  i_priority=None  i=0 A  i_nominal_specify=off  i_nominal_value=1  i_nominal_unit=A  v_specify=off  v_priority=None  v=0 V  v_nominal_specify=off  v_nominal_value=1  v_nominal_unit=V  vc_specify=off  vc_priority=High  vc=0 V  vc_nominal_specify=off  vc_nominal_value=1  vc_nominal_unit=V
  Resistor : fl_lib/Electrical/Electrical Elements/Resistor  R=Rsnu Ohm  i_specify=off  i_priority=None  i=0 A  i_nominal_specify=off  i_nominal_value=1  i_nominal_unit=A  v_specify=off  v_priority=None  v=0 V  v_nominal_specify=off  v_nominal_value=1  v_nominal_unit=V
  + : PMIOPort  Side=Left
  - : PMIOPort  Port=2  Side=Right
  connections:
  Resistor/LConn1 -- Capacitor/RConn1
  Capacitor/LConn1 -- +/RConn1
  Resistor/RConn1 -- -/RConn1

== system MATE_9LevelDrive_LowHarmonicRectifier/Diode Bridge with snubber8/RCsnuber5 ==
  Capacitor : fl_lib/Electrical/Electrical Elements/Capacitor  c=Csnu F  r=0 Ohm  g=0 1/Ohm  i_specify=off  i_priority=None  i=0 A  i_nominal_specify=off  i_nominal_value=1  i_nominal_unit=A  v_specify=off  v_priority=None  v=0 V  v_nominal_specify=off  v_nominal_value=1  v_nominal_unit=V  vc_specify=off  vc_priority=High  vc=0 V  vc_nominal_specify=off  vc_nominal_value=1  vc_nominal_unit=V
  Resistor : fl_lib/Electrical/Electrical Elements/Resistor  R=Rsnu Ohm  i_specify=off  i_priority=None  i=0 A  i_nominal_specify=off  i_nominal_value=1  i_nominal_unit=A  v_specify=off  v_priority=None  v=0 V  v_nominal_specify=off  v_nominal_value=1  v_nominal_unit=V
  + : PMIOPort  Side=Left
  - : PMIOPort  Port=2  Side=Right
  connections:
  Resistor/RConn1 -- -/RConn1
  Capacitor/LConn1 -- +/RConn1
  Resistor/LConn1 -- Capacitor/RConn1

== system MATE_9LevelDrive_LowHarmonicRectifier/Diode Bridge with snubber9/RCsnuber ==
  Capacitor : fl_lib/Electrical/Electrical Elements/Capacitor  c=Csnu F  r=0 Ohm  g=0 1/Ohm  i_specify=off  i_priority=None  i=0 A  i_nominal_specify=off  i_nominal_value=1  i_nominal_unit=A  v_specify=off  v_priority=None  v=0 V  v_nominal_specify=off  v_nominal_value=1  v_nominal_unit=V  vc_specify=off  vc_priority=High  vc=0 V  vc_nominal_specify=off  vc_nominal_value=1  vc_nominal_unit=V
  Resistor : fl_lib/Electrical/Electrical Elements/Resistor  R=Rsnu Ohm  i_specify=off  i_priority=None  i=0 A  i_nominal_specify=off  i_nominal_value=1  i_nominal_unit=A  v_specify=off  v_priority=None  v=0 V  v_nominal_specify=off  v_nominal_value=1  v_nominal_unit=V
  + : PMIOPort  Side=Left
  - : PMIOPort  Port=2  Side=Right
  connections:
  Resistor/LConn1 -- Capacitor/RConn1
  Capacitor/LConn1 -- +/RConn1
  Resistor/RConn1 -- -/RConn1

== system MATE_9LevelDrive_LowHarmonicRectifier/Diode Bridge with snubber9/RCsnuber1 ==
  Capacitor : fl_lib/Electrical/Electrical Elements/Capacitor  c=Csnu F  r=0 Ohm  g=0 1/Ohm  i_specify=off  i_priority=None  i=0 A  i_nominal_specify=off  i_nominal_value=1  i_nominal_unit=A  v_specify=off  v_priority=None  v=0 V  v_nominal_specify=off  v_nominal_value=1  v_nominal_unit=V  vc_specify=off  vc_priority=High  vc=0 V  vc_nominal_specify=off  vc_nominal_value=1  vc_nominal_unit=V
  Resistor : fl_lib/Electrical/Electrical Elements/Resistor  R=Rsnu Ohm  i_specify=off  i_priority=None  i=0 A  i_nominal_specify=off  i_nominal_value=1  i_nominal_unit=A  v_specify=off  v_priority=None  v=0 V  v_nominal_specify=off  v_nominal_value=1  v_nominal_unit=V
  + : PMIOPort  Side=Left
  - : PMIOPort  Port=2  Side=Right
  connections:
  Resistor/RConn1 -- -/RConn1
  Capacitor/LConn1 -- +/RConn1
  Resistor/LConn1 -- Capacitor/RConn1

== system MATE_9LevelDrive_LowHarmonicRectifier/Diode Bridge with snubber9/RCsnuber2 ==
  Capacitor : fl_lib/Electrical/Electrical Elements/Capacitor  c=Csnu F  r=0 Ohm  g=0 1/Ohm  i_specify=off  i_priority=None  i=0 A  i_nominal_specify=off  i_nominal_value=1  i_nominal_unit=A  v_specify=off  v_priority=None  v=0 V  v_nominal_specify=off  v_nominal_value=1  v_nominal_unit=V  vc_specify=off  vc_priority=High  vc=0 V  vc_nominal_specify=off  vc_nominal_value=1  vc_nominal_unit=V
  Resistor : fl_lib/Electrical/Electrical Elements/Resistor  R=Rsnu Ohm  i_specify=off  i_priority=None  i=0 A  i_nominal_specify=off  i_nominal_value=1  i_nominal_unit=A  v_specify=off  v_priority=None  v=0 V  v_nominal_specify=off  v_nominal_value=1  v_nominal_unit=V
  + : PMIOPort  Side=Left
  - : PMIOPort  Port=2  Side=Right
  connections:
  Resistor/LConn1 -- Capacitor/RConn1
  Capacitor/LConn1 -- +/RConn1
  Resistor/RConn1 -- -/RConn1

== system MATE_9LevelDrive_LowHarmonicRectifier/Diode Bridge with snubber9/RCsnuber3 ==
  Capacitor : fl_lib/Electrical/Electrical Elements/Capacitor  c=Csnu F  r=0 Ohm  g=0 1/Ohm  i_specify=off  i_priority=None  i=0 A  i_nominal_specify=off  i_nominal_value=1  i_nominal_unit=A  v_specify=off  v_priority=None  v=0 V  v_nominal_specify=off  v_nominal_value=1  v_nominal_unit=V  vc_specify=off  vc_priority=High  vc=0 V  vc_nominal_specify=off  vc_nominal_value=1  vc_nominal_unit=V
  Resistor : fl_lib/Electrical/Electrical Elements/Resistor  R=Rsnu Ohm  i_specify=off  i_priority=None  i=0 A  i_nominal_specify=off  i_nominal_value=1  i_nominal_unit=A  v_specify=off  v_priority=None  v=0 V  v_nominal_specify=off  v_nominal_value=1  v_nominal_unit=V
  + : PMIOPort  Side=Left
  - : PMIOPort  Port=2  Side=Right
  connections:
  Resistor/RConn1 -- -/RConn1
  Capacitor/LConn1 -- +/RConn1
  Resistor/LConn1 -- Capacitor/RConn1

== system MATE_9LevelDrive_LowHarmonicRectifier/Diode Bridge with snubber9/RCsnuber4 ==
  Capacitor : fl_lib/Electrical/Electrical Elements/Capacitor  c=Csnu F  r=0 Ohm  g=0 1/Ohm  i_specify=off  i_priority=None  i=0 A  i_nominal_specify=off  i_nominal_value=1  i_nominal_unit=A  v_specify=off  v_priority=None  v=0 V  v_nominal_specify=off  v_nominal_value=1  v_nominal_unit=V  vc_specify=off  vc_priority=High  vc=0 V  vc_nominal_specify=off  vc_nominal_value=1  vc_nominal_unit=V
  Resistor : fl_lib/Electrical/Electrical Elements/Resistor  R=Rsnu Ohm  i_specify=off  i_priority=None  i=0 A  i_nominal_specify=off  i_nominal_value=1  i_nominal_unit=A  v_specify=off  v_priority=None  v=0 V  v_nominal_specify=off  v_nominal_value=1  v_nominal_unit=V
  + : PMIOPort  Side=Left
  - : PMIOPort  Port=2  Side=Right
  connections:
  Resistor/RConn1 -- -/RConn1
  Capacitor/LConn1 -- +/RConn1
  Resistor/LConn1 -- Capacitor/RConn1

== system MATE_9LevelDrive_LowHarmonicRectifier/Diode Bridge with snubber9/RCsnuber5 ==
  Capacitor : fl_lib/Electrical/Electrical Elements/Capacitor  c=Csnu F  r=0 Ohm  g=0 1/Ohm  i_specify=off  i_priority=None  i=0 A  i_nominal_specify=off  i_nominal_value=1  i_nominal_unit=A  v_specify=off  v_priority=None  v=0 V  v_nominal_specify=off  v_nominal_value=1  v_nominal_unit=V  vc_specify=off  vc_priority=High  vc=0 V  vc_nominal_specify=off  vc_nominal_value=1  vc_nominal_unit=V
  Resistor : fl_lib/Electrical/Electrical Elements/Resistor  R=Rsnu Ohm  i_specify=off  i_priority=None  i=0 A  i_nominal_specify=off  i_nominal_value=1  i_nominal_unit=A  v_specify=off  v_priority=None  v=0 V  v_nominal_specify=off  v_nominal_value=1  v_nominal_unit=V
  + : PMIOPort  Side=Left
  - : PMIOPort  Port=2  Side=Right
  connections:
  Resistor/LConn1 -- Capacitor/RConn1
  Capacitor/LConn1 -- +/RConn1
  Resistor/RConn1 -- -/RConn1

== system MATE_9LevelDrive_LowHarmonicRectifier/ModulationSimulink/9-level inverter ctrl3 simulink ==
  signal : Inport
  carrier : Inport  Port=2
  Carriers Generator : Subsystem
  Mux3 : Mux  Inputs=16
  rte1 : Subsystem
  rte2 : Subsystem
  rte3 : Subsystem
  rte4 : Subsystem
  duty : Outport  VectorParamsAs1DForOutWhenUnconnected=off
  wires:
  signal/1 -> rte1/1(in), rte4/1(in), rte3/1(in), rte2/1(in)
  rte2/1(1) -> Mux3/1
  rte2/2(2) -> Mux3/2
  rte2/3(3) -> Mux3/3
  rte2/4(4) -> Mux3/4
  rte1/1(1) -> Mux3/5
  rte1/2(2) -> Mux3/6
  rte1/3(3) -> Mux3/7
  rte1/4(4) -> Mux3/8
  rte3/1(1) -> Mux3/9
  rte3/2(2) -> Mux3/10
  rte3/3(3) -> Mux3/11
  rte3/4(4) -> Mux3/12
  Mux3/1 -> duty/1
  carrier/1 -> Carriers Generator/1(c)
  Carriers Generator/8(C4-) -> rte2/3(c-)
  Carriers Generator/1(C4+) -> rte2/2(c+)
  Carriers Generator/2(C3+) -> rte1/2(c+)
  Carriers Generator/7(C3-) -> rte1/3(c-)
  Carriers Generator/3(C2+) -> rte3/2(c+)
  Carriers Generator/6(C2-) -> rte3/3(c-)
  Carriers Generator/4(C+) -> rte4/2(c+)
  rte4/1(1) -> Mux3/13
  rte4/2(2) -> Mux3/14
  rte4/3(3) -> Mux3/15
  rte4/4(4) -> Mux3/16
  Carriers Generator/5(C-) -> rte4/3(c-)

== system MATE_9LevelDrive_LowHarmonicRectifier/ModulationSimulink/9-level inverter ctrl3 simulink1 ==
  signal : Inport
  carrier : Inport  Port=2
  Carriers Generator : Subsystem
  Mux3 : Mux  Inputs=16
  rte1 : Subsystem
  rte2 : Subsystem
  rte3 : Subsystem
  rte4 : Subsystem
  duty : Outport  VectorParamsAs1DForOutWhenUnconnected=off
  wires:
  Carriers Generator/5(C-) -> rte4/3(c-)
  rte4/4(4) -> Mux3/16
  rte4/3(3) -> Mux3/15
  rte4/2(2) -> Mux3/14
  rte4/1(1) -> Mux3/13
  Carriers Generator/4(C+) -> rte4/2(c+)
  Carriers Generator/6(C2-) -> rte3/3(c-)
  Carriers Generator/3(C2+) -> rte3/2(c+)
  Carriers Generator/7(C3-) -> rte1/3(c-)
  Carriers Generator/2(C3+) -> rte1/2(c+)
  Carriers Generator/1(C4+) -> rte2/2(c+)
  Carriers Generator/8(C4-) -> rte2/3(c-)
  carrier/1 -> Carriers Generator/1(c)
  Mux3/1 -> duty/1
  rte3/4(4) -> Mux3/12
  rte3/3(3) -> Mux3/11
  rte3/2(2) -> Mux3/10
  rte3/1(1) -> Mux3/9
  rte1/4(4) -> Mux3/8
  rte1/3(3) -> Mux3/7
  rte1/2(2) -> Mux3/6
  rte1/1(1) -> Mux3/5
  rte2/4(4) -> Mux3/4
  rte2/3(3) -> Mux3/3
  rte2/2(2) -> Mux3/2
  rte2/1(1) -> Mux3/1
  signal/1 -> rte2/1(in), rte3/1(in), rte4/1(in), rte1/1(in)

== system MATE_9LevelDrive_LowHarmonicRectifier/ModulationSimulink/9-level inverter ctrl3 simulink2 ==
  signal : Inport
  carrier : Inport  Port=2
  Carriers Generator : Subsystem
  Mux3 : Mux  Inputs=16
  rte1 : Subsystem
  rte2 : Subsystem
  rte3 : Subsystem
  rte4 : Subsystem
  duty : Outport  VectorParamsAs1DForOutWhenUnconnected=off
  wires:
  signal/1 -> rte1/1(in), rte4/1(in), rte3/1(in), rte2/1(in)
  rte2/1(1) -> Mux3/1
  rte2/2(2) -> Mux3/2
  rte2/3(3) -> Mux3/3
  rte2/4(4) -> Mux3/4
  rte1/1(1) -> Mux3/5
  rte1/2(2) -> Mux3/6
  rte1/3(3) -> Mux3/7
  rte1/4(4) -> Mux3/8
  rte3/1(1) -> Mux3/9
  rte3/2(2) -> Mux3/10
  rte3/3(3) -> Mux3/11
  rte3/4(4) -> Mux3/12
  Mux3/1 -> duty/1
  carrier/1 -> Carriers Generator/1(c)
  Carriers Generator/8(C4-) -> rte2/3(c-)
  Carriers Generator/1(C4+) -> rte2/2(c+)
  Carriers Generator/2(C3+) -> rte1/2(c+)
  Carriers Generator/7(C3-) -> rte1/3(c-)
  Carriers Generator/3(C2+) -> rte3/2(c+)
  Carriers Generator/6(C2-) -> rte3/3(c-)
  Carriers Generator/4(C+) -> rte4/2(c+)
  rte4/1(1) -> Mux3/13
  rte4/2(2) -> Mux3/14
  rte4/3(3) -> Mux3/15
  rte4/4(4) -> Mux3/16
  Carriers Generator/5(C-) -> rte4/3(c-)

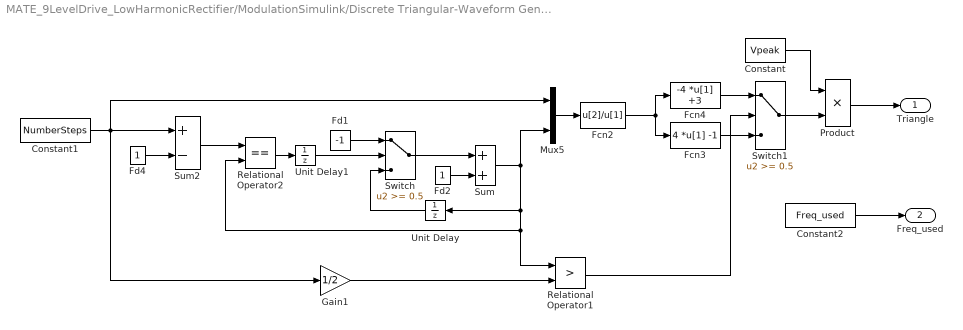
== system MATE_9LevelDrive_LowHarmonicRectifier/ModulationSimulink/Discrete Triangular-Waveform Generator ==
  Constant : Constant  Value=Vpeak
  Constant1 : Constant  Value=NumberSteps
  Constant2 : Constant  Value=Freq_used
  Fcn2 : Fcn  Expr=u[2]/u[1]
  Fcn3 : Fcn  Expr=4 *u[1] -1
  Fcn4 : Fcn  Expr=-4 *u[1] +3
  Fd1 : Constant  Value=-1
  Fd2 : Constant
  Fd4 : Constant
  Gain1 : Gain  Gain=1/2  SaturateOnIntegerOverflow=on  OutDataTypeStr=Inherit: Same as input  ParamDataTypeStr=Inherit: Same as input
  Mux5 : Mux  Inputs=2
  Product : Product  InputSameDT=on  SaturateOnIntegerOverflow=on  OutDataTypeStr=Inherit: Same as first input
  Relational Operator1 : RelationalOperator  Operator=>
  Relational Operator2 : RelationalOperator  Operator===
  Sum : Sum  InputSameDT=on  SaturateOnIntegerOverflow=on  OutDataTypeStr=Inherit: Same as first input
  Sum2 : Sum  Inputs=+-  InputSameDT=on  SaturateOnIntegerOverflow=on  OutDataTypeStr=Inherit: Same as first input
  Switch : Switch  Threshold=0.5
  Switch1 : Switch  Threshold=0.5
  Unit Delay : UnitDelay  SampleTime=Ts  HasFrameUpgradeWarning=on
  Unit Delay1 : UnitDelay  SampleTime=Ts  HasFrameUpgradeWarning=on
  Triangle : Outport  InitialOutput=0  VectorParamsAs1DForOutWhenUnconnected=off
  Freq_used : Outport  Port=2  InitialOutput=0  VectorParamsAs1DForOutWhenUnconnected=off
  wires:
  Constant2/1 -> Freq_used/1
  Relational Operator1/1 -> Switch1/2
  Gain1/1 -> Relational Operator1/2
  Fcn3/1 -> Switch1/3
  Fcn4/1 -> Switch1/1
  Mux5/1 -> Fcn2/1
  Fcn2/1 -> Fcn3/1, Fcn4/1
  Sum/1 -> Mux5/2, Relational Operator1/1, Relational Operator2/2, Unit Delay/1
  Constant1/1 -> Gain1/1, Mux5/1, Sum2/1
  Sum2/1 -> Relational Operator2/1
  Relational Operator2/1 -> Unit Delay1/1
  Unit Delay1/1 -> Switch/2
  Unit Delay/1 -> Switch/3
  Fd1/1 -> Switch/1
  Fd2/1 -> Sum/2
  Switch/1 -> Sum/1
  Fd4/1 -> Sum2/2
  Constant/1 -> Product/1
  Switch1/1 -> Product/2
  Product/1 -> Triangle/1
